simulink model "Ex4_1_Battery_DCMotor_SoCEstimation"  (R2024b)
settings: Solver=VariableStepAuto  StartTime=0.0  StopTime=3600*3  RelTol=1e-3
undefined symbols (not defined in the file): Ion, Lithium
libraries: spsBatteryLib x1, spsCurrentMeasurementLib x1, spsDCMachineLib x1, sps_lib x1
settings Model: Creator=balaj  LastModifiedBy=balaj

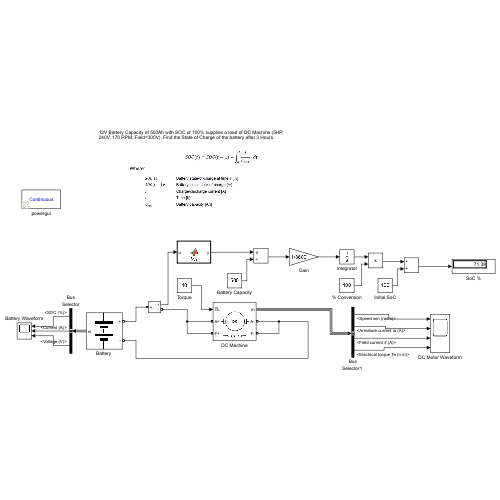
[thumbnail: Simulink's stored preview of the top-level diagram]
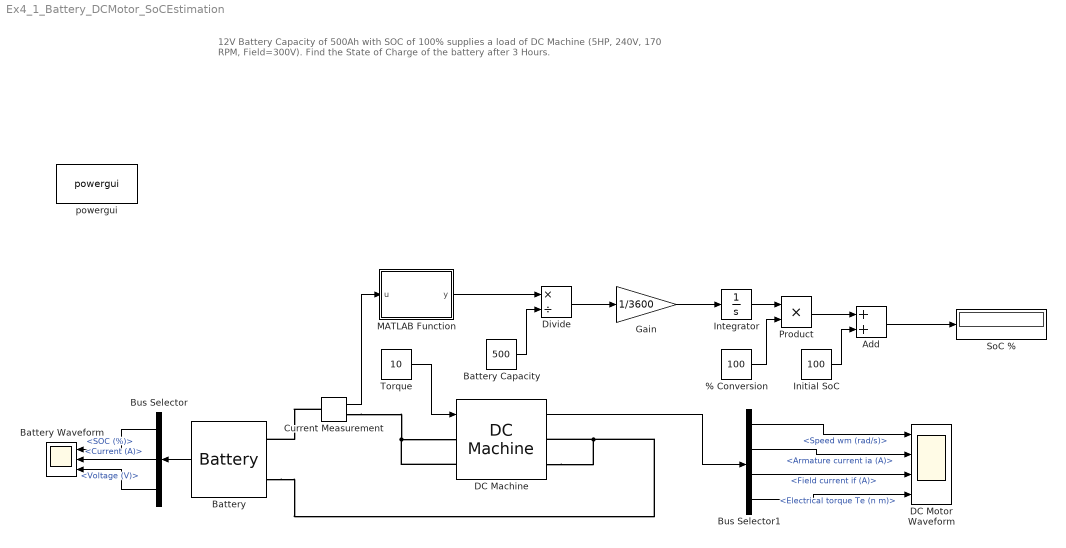
== system Ex4_1_Battery_DCMotor_SoCEstimation ==
  note: 12V Battery Capacity of 500Ah with SOC of 100% supplies a load of DC Machine (5HP, 240V, 170 RPM, Field=300V). Find the State of Charge of the battery after 3 Hours.
  % Conversion : Constant  Value=100
  Add : Sum
  "Battery " : spsBatteryLib/Battery  BatType=Lithium-Ion  NomV=12  NomQ=500  SOC=100  Batt_Tr=30  PresetModel=on  MaxQ=500  MinV=9  FullV=13.9678  Dis_rate=217.3913  R=0.00024  Normal_OP=452.1739  expZone="[12.9646      24.5652]"
  Battery Capacity : Constant  Value=500
  Battery Waveform : Scope  NumInputPorts=3
  Bus Selector : BusSelector  OutputSignals=SOC (%),Current (A),Voltage (V)
  "Bus Selector1 " : BusSelector  OutputSignals=Speed wm (rad/s),Armature current ia (A),Field current if (A),Electrical torque Te (n m)
  Current Measurement : spsCurrentMeasurementLib/Current Measurement  PhasorSimulation=off  OutputType=Complex  PSBequivalent=0
  DC Machine : spsDCMachineLib/DC Machine  PresetModel=01: 5HP 240V 1750RPM Field:300V  MechanicalLoad=Torque TL  FieldType=Wound  ShowDetailedParameters=on  MeasurementBus=off  RLa=[2.581 0.028]  RLf=[281.2 156]  Laf=0.9483  MachineConstant=Torque constant (N.m/A)  Ke=1.8  Kt=1.8  J=0.02215  Bm=0.002953  Tf=0.5161  w0=1  Ifinit=0  TsPowergui=0  TsBlock=-1
  DC Motor Waveform : Scope  NumInputPorts=4
  Divide : Product  Inputs=*/
  Gain : Gain  Gain=1/3600
  Initial SoC : Constant  Value=100
  Integrator : Integrator
  MATLAB Function : MATLAB Function  TreatAsAtomicUnit=on
  Product : Product
  SoC % : Display
  Torque : Constant  Value=10
  powergui : sps_lib/powergui  Priority=1  SimulationMode=Continuous  SampleTime=50e-6  frequency=60  Iterations=50  frequencyindice=0  Pbase=100e6  ErrMax=1e-4  UnitsV=kV  UnitsW=MW  buscounter=0  FunctionMessages=off  echomessages=off  EnableUseOfTLC=off  CurrentSourceSwitches=off  DisableSnubberDevices=off  DisableRonSwitches=off  DisableVfSwitches=off  DisplayEquations=off  AutomaticDiscreteSolvers=off  SolverType=Tustin/Backward Euler (TBE)  Interpol=off  ExternalGateDelay=off  methode=off  Ts=100  x0status=blocks  SPID=on  SwTol=0  HookPort=off  NonlinearTolerance=1e-4  nMaxIteration=100  ContinueOnMaxIteration=off  RestoreLinks=warning  ResistiveCurrentMeasurement=off  Frange=[0:2:500]  Ylog=off  Xlog=on  ShowGrid=off  save=off  variable=ZData  structure=0  ZoomFFT=off  StartTime=0.0  cycles=1  DisplayStyle=1  fundamental=60  FreqAxis=off  MaxFrequency=1000  frequencyindicesteady=1  RmsSteady=1  display=off
  wires:
  Torque/1 -> DC Machine/1
  "Battery "/1 -> Bus Selector/1
  Bus Selector/1 -> Battery Waveform/1  "<SOC (%)>"
  Bus Selector/2 -> Battery Waveform/2  "<Current (A)>"
  Bus Selector/3 -> Battery Waveform/3  "<Voltage (V)>"
  Current Measurement/1 -> MATLAB Function/1(u)
  MATLAB Function/1(y) -> Divide/1
  Battery Capacity/1 -> Divide/2
  Divide/1 -> Gain/1
  Gain/1 -> Integrator/1
  Integrator/1 -> Product/1
  % Conversion/1 -> Product/2
  Product/1 -> Add/1
  Initial SoC/1 -> Add/2
  Add/1 -> SoC %/1
  DC Machine/1 -> "Bus Selector1 "/1
  "Bus Selector1 "/1 -> DC Motor Waveform/1  "<Speed wm (rad/s)>"
  "Bus Selector1 "/2 -> DC Motor Waveform/2  "<Armature current ia (A)>"
  "Bus Selector1 "/3 -> DC Motor Waveform/3  "<Field current if (A)>"
  "Bus Selector1 "/4 -> DC Motor Waveform/4  "<Electrical torque Te (n m)>"
  connections:
  "Battery "/LConn2 -- DC Machine/RConn2 -- DC Machine/RConn1
  Current Measurement/LConn1 -- "Battery "/LConn1
  Current Measurement/RConn1 -- DC Machine/LConn1 -- DC Machine/LConn2

== matlab function Ex4_1_Battery_DCMotor_SoCEstimation/MATLAB Function ==
  data: u input; y output
function y = fcn(u)

y = -u;
